simulink model "torch"  (R2024a)
settings: Solver=FixedStepAuto  StartTime=0.0  StopTime=50  FixedStep=framePeriod_s  RelTol=1e-3
undefined symbols (not defined in the file): Aircraft, DiscIntNeverNeededParam, framePeriod_s, frameRate_hz, magnitude
libraries: simulink x35, slpidlib x11, dspmathops x1, simulink_extras x1
(part 4 of 4)

== matlab function torch/OUTER_TO_INNER_CONV/ tilt_limiter ==
  data: thrust_vector_raw input size=[3,1]; limited_vector output size=[3,1]
 function limited_vector = tilt_limiter (thrust_vector_raw)
    % Modify the acceleration command so that the tilt is within limit
    % It should also maintain the vertical acceleration command
    % Input:    
    %           thrust_vector_raw - raw acceleration command, can be anything
    %           angle_lim_deg - lean angle limit
    % Output:   
    %           limited_vector - limited acceleration vector
    temp = single(dot(thrust_vector_raw/norm(thrust_vector_raw),[0 0 -1]));
    if temp >= 0.9659 % This constant is precomputed from cosd(15)
        limited_vector = thrust_vector_raw;
    else
        a_z_new = thrust_vector_raw(3); 
        r = abs(a_z_new * 0.2679); % This constant is precomputed from tand(15)
        sqrt_temp = single(sqrt(thrust_vector_raw(1)^2 + thrust_vector_raw(2)^2));
        cos_phi = thrust_vector_raw(2) / sqrt_temp;
        sin_phi = thrust_vector_raw(1) / sqrt_temp;
        a_x_new = r * sin_phi;
        a_y_new = r * cos_phi;
        limited_vector = [a_x_new; a_y_new; a_z_new];
    end
end

== matlab function torch/command selection/mode_norm1/remap ==
  data: raw_in input; norm_out output; in_min input; in_max input; out_min input; out_max input
function norm_out = remap(raw_in,in_min,in_max,out_min,out_max)
norm_out = (raw_in - in_min) * (out_max - out_min)/(in_max-in_min) + out_min;

== matlab function torch/OUTER_TO_INNER_CONV/thrust_limit ==
  data: thrust_vector_raw input size=[3,1]; limited_vector output size=[3,1]; max_thrust input
function limited_vector = limit_thrust(thrust_vector_raw, max_thrust)
    % Limit the acceleration command to the max thrust achievable by the
    % aircraft. Should prioritize vertical thrust
    % Input:
    %           thrust_vector_raw - raw acceleration command
    %           max_thrust - max thrust by aircraft. In term of G
    limited_vector = single(thrust_vector_raw);
    mag = single(norm(thrust_vector_raw));
    % Ignore if the acc_cmd is already achieble
    if mag < max_thrust
        limited_vector = thrust_vector_raw;
    else
        if thrust_vector_raw(3) < -max_thrust
            limited_vector(3) = -max_thrust;
        end
        hor_acc = sqrt(max_thrust^2 - limited_vector(3)^2);
        limited_vector(1) = thrust_vector_raw(1) * hor_acc/mag;
        limited_vector(2) = thrust_vector_raw(2) * hor_acc/mag;
    end
    limited_vector = single(limited_vector);
end

== matlab function torch/POS_HOLD_input_conversion/Circular constraint ==
  data: x output; x_in input; y output; y_in input
function [x,y] = circular_limit(x_in, y_in)
    % Normalize square [-1,1] to unit circular limit
    r = sqrt(x_in.^2 + y_in.^2);
    if r <= 1
        x = x_in;
        y = y_in;
    else
        x = x_in ./ r;
        y = y_in ./ r;
    end
end

== matlab function torch/Stab_input_conversion/Circular constraint ==
  data: x output; x_in input; y output; y_in input
function [x,y] = circular_limit(x_in, y_in)
    % Normalize square [-1,1] to unit circular limit
    r = sqrt(x_in^2 + y_in^2);
    if r <= 1
        x = x_in;
        y = y_in;
    else
        x = x_in / r;
        y = y_in / r;
    end
end

== matlab function torch/OUTER_TO_INNER_CONV/tilt_command_calculation ==
  data: thrust_vector_ned input; phi_rad output; psi_rad input; theta_rad output
function [phi_rad, theta_rad] = calc_tilt (thrust_vector_ned, psi_rad)
    % Calculate the pitch and roll of the aircraft required to tilt the
    % thrust vector to match independent of its heading. 
    % Input:    
    %           thrust_vector_ned - commanded acceleration vector in NED
    %           frame. Should be unit vector
    %           psi_rad - the current heading angle of the aircraft. 
    % Output:   
    %           phi_rad, theta_rad - calculated pitch and roll angle
    %           requires for the thrust vector to match with the commanded
    %           inertial vector
    thrust_vector_ned = thrust_vector_ned/norm(thrust_vector_ned);
    cpsi = single(cos(psi_rad));
    spsi = single(sin(psi_rad));
    theta_num = cpsi * thrust_vector_ned(1) + spsi * thrust_vector_ned(2);
    theta_denum = thrust_vector_ned(3);
    theta_rad = single(atan2(theta_num, theta_denum)) + pi;
    if theta_rad > pi
        theta_rad = theta_rad - 2*pi;
    end
    ctheta = single(cos(theta_rad));
    stheta = single(sin(theta_rad));
    phi_num = stheta * cpsi * thrust_vector_ned(1) + ...
        stheta * spsi * thrust_vector_ned(2) + ctheta * thrust_vector_ned(3);
    phi_denum = spsi * thrust_vector_ned(1) - cpsi * thrust_vector_ned(2);
    phi_rad = single(atan2(phi_denum, phi_num)) + pi;
    if phi_rad > pi
        phi_rad = phi_rad - 2*pi;
    end
    theta_rad = single(theta_rad);
    phi_rad = single(phi_rad);
end

== matlab function torch/OUTER_TO_INNER_CONV/calc_body_throttle ==
  data: raw_thrust_vector input size=[3,1]; throttle output; hover_thr input; max_g_thrust input; gain input
function throttle = calc_body_throttle(raw_thrust_vector, hover_thr, max_g_thrust,gain)
    mag = norm(raw_thrust_vector);
    throttle = hover_thr + gain * (1 - hover_thr)*(mag - 1)/(max_g_thrust - 1);
    throttle = single(throttle);
end

== matlab function torch/command selection/yaw_norm_deadband/remap_with_deadband ==
  data: raw_in input; norm_out output; in_min input; in_max input; out_min input; out_max input; deadband input
function norm_out = remap_deadband(raw_in, in_min, in_max, out_min, out_max, deadband)
in_avg = (in_min + in_max) / 2;
out_avg = (out_min + out_max) / 2;

in_deadband_range = (in_max - in_min) * deadband / 2;
in_deadband_low = in_avg - in_deadband_range;
in_deadband_hi = in_avg + in_deadband_range;

if raw_in < in_deadband_low
    norm_out = (raw_in - in_deadband_low) .* (out_max - out_avg)./(in_deadband_low - in_min) + out_avg;
elseif raw_in > in_deadband_low && raw_in < in_deadband_hi
    norm_out = out_avg;
else
    norm_out = (raw_in - in_deadband_hi) .* (out_max - out_avg)./(in_max - in_deadband_hi) + out_avg;
end

== matlab function torch/command selection/throttle_norm/remap ==
  data: raw_in input; norm_out output; in_min input; in_max input; out_min input; out_max input
function norm_out = remap(raw_in,in_min,in_max,out_min,out_max)
norm_out = (raw_in - in_min) * (out_max - out_min)/(in_max-in_min) + out_min;

== matlab function torch/POS_HOLD_input_conversion/pitch_norm_deadband/remap_with_deadband ==
  data: raw_in input; norm_out output; in_min input; in_max input; out_min input; out_max input; deadband input
function norm_out = remap_deadband(raw_in, in_min, in_max, out_min, out_max, deadband)
in_avg = (in_min + in_max) / 2;
out_avg = (out_min + out_max) / 2;

in_deadband_range = (in_max - in_min) * deadband / 2;
in_deadband_low = in_avg - in_deadband_range;
in_deadband_hi = in_avg + in_deadband_range;

if raw_in < in_deadband_low
    norm_out = (raw_in - in_deadband_low) .* (out_max - out_avg)./(in_deadband_low - in_min) + out_avg;
elseif raw_in > in_deadband_low && raw_in < in_deadband_hi
    norm_out = out_avg;
else
    norm_out = (raw_in - in_deadband_hi) .* (out_max - out_avg)./(in_max - in_deadband_hi) + out_avg;
end

== matlab function torch/command selection/roll_norm_deadband/remap_with_deadband ==
  data: raw_in input; norm_out output; in_min input; in_max input; out_min input; out_max input; deadband input
function norm_out = remap_deadband(raw_in, in_min, in_max, out_min, out_max, deadband)
in_avg = (in_min + in_max) / 2;
out_avg = (out_min + out_max) / 2;

in_deadband_range = (in_max - in_min) * deadband / 2;
in_deadband_low = in_avg - in_deadband_range;
in_deadband_hi = in_avg + in_deadband_range;

if raw_in < in_deadband_low
    norm_out = (raw_in - in_deadband_low) .* (out_max - out_avg)./(in_deadband_low - in_min) + out_avg;
elseif raw_in > in_deadband_low && raw_in < in_deadband_hi
    norm_out = out_avg;
else
    norm_out = (raw_in - in_deadband_hi) .* (out_max - out_avg)./(in_max - in_deadband_hi) + out_avg;
end

== matlab function torch/command selection/pitch_norm_deadband/remap_with_deadband ==
  data: raw_in input; norm_out output; in_min input; in_max input; out_min input; out_max input; deadband input
function norm_out = remap_deadband(raw_in, in_min, in_max, out_min, out_max, deadband)
in_avg = (in_min + in_max) / 2;
out_avg = (out_min + out_max) / 2;

in_deadband_range = (in_max - in_min) * deadband / 2;
in_deadband_low = in_avg - in_deadband_range;
in_deadband_hi = in_avg + in_deadband_range;

if raw_in < in_deadband_low
    norm_out = (raw_in - in_deadband_low) .* (out_max - out_avg)./(in_deadband_low - in_min) + out_avg;
elseif raw_in > in_deadband_low && raw_in < in_deadband_hi
    norm_out = out_avg;
else
    norm_out = (raw_in - in_deadband_hi) .* (out_max - out_avg)./(in_max - in_deadband_hi) + out_avg;
end

== matlab function torch/command selection/e_stop_norm/remap ==
  data: raw_in input; norm_out output; in_min input; in_max input; out_min input; out_max input
function norm_out = remap(raw_in,in_min,in_max,out_min,out_max)
norm_out = (raw_in - in_min) * (out_max - out_min)/(in_max-in_min) + out_min;
